simulink model "SF045A_HwAgSysArbn"  (R2013b)
settings: Solver=FixedStepDiscrete  SolverMode=SingleTasking  StartTime=0.0  StopTime=1  FixedStep=.002  RelTol=1e-3
values from neighbouring files (symbols this model uses):
  ARCHGLBPRM_2MILLISEC_SEC_F32 = DataDict.Constant    [SF045A_HwAgSysArbn_DataDict.m]
  ARCHGLBPRM_FLOATZEROTHD_ULS_F32 = DataDict.Constant    [SF045A_HwAgSysArbn_DataDict.m]
  ARCHGLBPRM_PIOVER180_ULS_F32 = DataDict.Constant    [SF045A_HwAgSysArbn_DataDict.m]
  CNVSECTOCNT_ULS_U32 = DataDict.Constant    [SF045A_HwAgSysArbn_DataDict.m]
  CNVTOMILLISEC_MILLISECPERCNT_F32 = DataDict.Constant    [SF045A_HwAgSysArbn_DataDict.m]
  FltInj_f32 = DataDict.Client    [SF045A_HwAgSysArbn_DataDict.m]
  FLTINJ_HWAGSYSARBN_HWAG = DataDict.Constant    [SF045A_HwAgSysArbn_DataDict.m]
  FLTINJ_HWAGSYSARBN_SERLCOMHWAG = DataDict.Constant    [SF045A_HwAgSysArbn_DataDict.m]
  HwAgCorrlnFlt = DataDict.NTC    [SF045A_HwAgSysArbn_DataDict.m]
  HwAgSnsrlsThdExcdd = DataDict.NTC    [SF045A_HwAgSysArbn_DataDict.m]
  HwAgSysArbnHwAgConf1Snsr = DataDict.Calibration    [SF045A_HwAgSysArbn_DataDict.m]
  HwAgSysArbnHwAgConf2Snsr = DataDict.Calibration    [SF045A_HwAgSysArbn_DataDict.m]
  HwAgSysArbnHwAgConfNoSnsr = DataDict.Calibration    [SF045A_HwAgSysArbn_DataDict.m]
  HwAgSysArbnHwAgCorrdCorrlnThd = DataDict.Calibration    [SF045A_HwAgSysArbn_DataDict.m]
  HwAgSysArbnHwAgCorrlnFailDebStep = DataDict.Calibration    [SF045A_HwAgSysArbn_DataDict.m]
  HwAgSysArbnHwAgCorrlnPassDebStep = DataDict.Calibration    [SF045A_HwAgSysArbn_DataDict.m]
  HwAgSysArbnHwAgCorrlnRng = DataDict.Calibration    [SF045A_HwAgSysArbn_DataDict.m]
  HwAgSysArbnHwAgSlewRate = DataDict.Calibration    [SF045A_HwAgSysArbn_DataDict.m]
  HwAgSysArbnHwAgSnsrlsCorrlnThd = DataDict.Calibration    [SF045A_HwAgSysArbn_DataDict.m]
  HwAgSysArbnHwAgSnsrlsKineThd = DataDict.Calibration    [SF045A_HwAgSysArbn_DataDict.m]
  HwAgSysArbnHwAgToMotAgCorrlnElpdTiLim = DataDict.Calibration    [SF045A_HwAgSysArbn_DataDict.m]
  HwAgSysArbnSerlComHwAgCorrdConf = DataDict.Calibration    [SF045A_HwAgSysArbn_DataDict.m]
  HwAgSysArbnSerlComHwAgSnsrlsConf = DataDict.Calibration    [SF045A_HwAgSysArbn_DataDict.m]
  HwAgSysArbnSlewRateTmr = DataDict.Calibration    [SF045A_HwAgSysArbn_DataDict.m]
  HWAGTHD_ULS_FLOAT32 = DataDict.Constant    [SF045A_HwAgSysArbn_DataDict.m]
  INVLDSRC_CNT_S08 = DataDict.Constant    [SF045A_HwAgSysArbn_DataDict.m]
  LRGSLEW_HWDEGPERSEC_F32 = DataDict.Constant    [SF045A_HwAgSysArbn_DataDict.m]
  NODEBSTEP_CNT_U16 = DataDict.Constant    [SF045A_HwAgSysArbn_DataDict.m]
  SLEWINPROGS_CNT_LGC = DataDict.Constant    [SF045A_HwAgSysArbn_DataDict.m]
  SLEWNOTINPROGS_CNT_LGC = DataDict.Constant    [SF045A_HwAgSysArbn_DataDict.m]
  SNSRDATASRCSELD_CNT_S08 = DataDict.Constant    [SF045A_HwAgSysArbn_DataDict.m]
  SNSRLSDATASRCSELD_CNT_S08 = DataDict.Constant    [SF045A_HwAgSysArbn_DataDict.m]
  SysGlbPrmSysKineRat = DataDict.ImprtdCal    [SF045A_HwAgSysArbn_DataDict.m]
  SysGlbPrmTorsBarStfn = DataDict.ImprtdCal    [SF045A_HwAgSysArbn_DataDict.m]
  ZEROTMR_MILLISEC_F32 = DataDict.Constant    [SF045A_HwAgSysArbn_DataDict.m]
undefined symbols (not defined in the file or in its folder): NtcSts1
libraries: NxtrLim x11, simulink x6, NxtrAbslt x6, Fil x3, autosarlib x2
(part 6 of 6)

== system SF045A_HwAgSysArbn/HwAgSysArbn/HwAgSysArbnPer1/HwAgArbn/VldtSnsrlsData/ThdExcdd/Kinematic Integrity/SetNtcSts ==
  note: Note:
      |
      | - "ISO Fault Debounce Design" Simulink block intent to use here for Simulation purpose only. Do not Code this block
  NtcNr : Inport
  NtcStInfo : Inport  Port=2
  NtcSts : Inport  Port=3
  DebStep : Inport  Port=4
  CopyRight2 : Subsystem  Description=|  mask(Copyright Information){none=on}
      | Copyright info block.                                               
      |                                                                     
      | Place copyright information at the top of every subsystem in design.
      mask prompts: none "No parameters"
      mask help: Place copyright information at the top of every subsystem in design.
      mask Display:
      | NxtrConf = 'Nexteer Confidential';
      | 
      | sys = bdroot; %handle for the current model ("system")
      | first = get_param(sys,'Created');
      | if(isempty(first))
      |     first = datestr(now,'yyyy');
      | else
      |     first = first(end-3:end);  %year is last four digits
      | end
      | 
      | last = get_param(sys,'LastModifiedDate');
      | if isempty(last)
      |     last = datestr(now,'yyyy');
      | else
      |     last = last(end-3:end);
      | end
      | 
      | if strcmp(first,last)
      |     fprintf('%s -- Copyright %s Nexteer',NxtrConf,first)
      | else
      |     fprintf('%s -- %s%s- %s Nexteer',NxtrConf,char(169),first,last)
      | end
  Data Store Write : DataStoreWrite  DataStoreName=NtcQlfr
  Data Store Write1 : DataStoreWrite  DataStoreName=NtcQlfrHwAgSnsrlsThdExcd
  Data Store Write2 : DataStoreWrite  DataStoreName=NtcStInfoHwAgSnsrlsThdExcd
  Data Store Write3 : DataStoreWrite  DataStoreName=NtcStsHwAgSnsrlsThdExcd
  Data Type Conversion : DataTypeConversion  OutDataTypeStr=Enum: SigQlfr1
  Data Type Conversion1 : DataTypeConversion  OutDataTypeStr=uint8
  Ground : Ground
  ISO Fault Debounce Design : Stateflow chart  TreatAsAtomicUnit=on
      settings: AttributesFormatString=|
      | Simulation Purpose Only.
      | Do Not Code this block
      | Diagnostic Manager Owns this requirement
  Terminator : Terminator
  Terminator1 : Terminator
  wires:
  Data Type Conversion1/1 -> Data Store Write2/1
  NtcStInfo/1 -> Terminator1/1, Data Type Conversion1/1
  NtcSts/1 -> ISO Fault Debounce Design/1(NtcSts), Data Store Write3/1
  Data Type Conversion/1 -> Data Store Write/1, Data Store Write1/1
  Ground/1 -> ISO Fault Debounce Design/3(SvcClr)
  ISO Fault Debounce Design/1(Qualifier) -> Data Type Conversion/1
  DebStep/1 -> ISO Fault Debounce Design/2(DebStep)
  NtcNr/1 -> Terminator/1

== system SF045A_HwAgSysArbn/HwAgSysArbn/HwAgSysArbnPer1/HwAgArbn/HwAgVelSeriCom/ChkCorrln/SetCorrlFltNtc/SetCorrlFltNtc/SetNtcSts ==
  note: Note:
      |
      | - "ISO Fault Debounce Design" Simulink block intent to use here for Simulation purpose only. Do not Code this block
  NtcNr : Inport
  NtcStInfo : Inport  Port=2
  NtcSts : Inport  Port=3
  DebStep : Inport  Port=4
  CopyRight2 : Subsystem  Description=|  mask(Copyright Information){none=on}
      | Copyright info block.                                               
      |                                                                     
      | Place copyright information at the top of every subsystem in design.
      mask prompts: none "No parameters"
      mask help: Place copyright information at the top of every subsystem in design.
      mask Display:
      | NxtrConf = 'Nexteer Confidential';
      | 
      | sys = bdroot; %handle for the current model ("system")
      | first = get_param(sys,'Created');
      | if(isempty(first))
      |     first = datestr(now,'yyyy');
      | else
      |     first = first(end-3:end);  %year is last four digits
      | end
      | 
      | last = get_param(sys,'LastModifiedDate');
      | if isempty(last)
      |     last = datestr(now,'yyyy');
      | else
      |     last = last(end-3:end);
      | end
      | 
      | if strcmp(first,last)
      |     fprintf('%s -- Copyright %s Nexteer',NxtrConf,first)
      | else
      |     fprintf('%s -- %s%s- %s Nexteer',NxtrConf,char(169),first,last)
      | end
  Data Store Write : DataStoreWrite  DataStoreName=NtcQlfr
  Data Store Write1 : DataStoreWrite  DataStoreName=NtcQlfrHwAgToMotAgCorrln
  Data Store Write2 : DataStoreWrite  DataStoreName=NtcStInfoHwAgToMotAgCorrln
  Data Store Write3 : DataStoreWrite  DataStoreName=NtcStsHwAgToMotAgCorrln
  Data Type Conversion : DataTypeConversion  OutDataTypeStr=Enum: SigQlfr1
  Data Type Conversion1 : DataTypeConversion  OutDataTypeStr=uint8
  Ground : Ground
  ISO Fault Debounce Design : Stateflow chart  TreatAsAtomicUnit=on
      settings: AttributesFormatString=|
      | Simulation Purpose Only.
      | Do Not Code this block
      | Diagnostic Manager Owns this requirement
  Terminator : Terminator
  Terminator1 : Terminator
  wires:
  Data Type Conversion1/1 -> Data Store Write2/1
  NtcStInfo/1 -> Terminator1/1, Data Type Conversion1/1
  NtcSts/1 -> ISO Fault Debounce Design/1(NtcSts), Data Store Write3/1
  Data Type Conversion/1 -> Data Store Write/1, Data Store Write1/1
  Ground/1 -> ISO Fault Debounce Design/3(SvcClr)
  ISO Fault Debounce Design/1(Qualifier) -> Data Type Conversion/1
  DebStep/1 -> ISO Fault Debounce Design/2(DebStep)
  NtcNr/1 -> Terminator/1

== system SF045A_HwAgSysArbn/HwAgSysArbn/HwAgSysArbnPer1/HwAgArbn/HwAgVelSeriCom/ChkCorrln/SetNtcPass/GetRefTmr100MicroSec32bit/CopyRight2 ==

== system SF045A_HwAgSysArbn/HwAgSysArbn/HwAgSysArbnPer1/HwAgArbn/HwAgVelSeriCom/ChkCorrln/SetNtcPass/SetNtcPass/SetNtcSts ==
  note: Note:
      |
      | - "ISO Fault Debounce Design" Simulink block intent to use here for Simulation purpose only. Do not Code this block
  NtcNr : Inport
  NtcStInfo : Inport  Port=2
  NtcSts : Inport  Port=3
  DebStep : Inport  Port=4
  CopyRight2 : Subsystem  Description=|  mask(Copyright Information){none=on}
      | Copyright info block.                                               
      |                                                                     
      | Place copyright information at the top of every subsystem in design.
      mask prompts: none "No parameters"
      mask help: Place copyright information at the top of every subsystem in design.
      mask Display:
      | NxtrConf = 'Nexteer Confidential';
      | 
      | sys = bdroot; %handle for the current model ("system")
      | first = get_param(sys,'Created');
      | if(isempty(first))
      |     first = datestr(now,'yyyy');
      | else
      |     first = first(end-3:end);  %year is last four digits
      | end
      | 
      | last = get_param(sys,'LastModifiedDate');
      | if isempty(last)
      |     last = datestr(now,'yyyy');
      | else
      |     last = last(end-3:end);
      | end
      | 
      | if strcmp(first,last)
      |     fprintf('%s -- Copyright %s Nexteer',NxtrConf,first)
      | else
      |     fprintf('%s -- %s%s- %s Nexteer',NxtrConf,char(169),first,last)
      | end
  Data Store Write : DataStoreWrite  DataStoreName=NtcQlfr
  Data Store Write1 : DataStoreWrite  DataStoreName=NtcQlfrHwAgToMotAgCorrln
  Data Store Write2 : DataStoreWrite  DataStoreName=NtcStInfoHwAgToMotAgCorrln
  Data Store Write3 : DataStoreWrite  DataStoreName=NtcStsHwAgToMotAgCorrln
  Data Type Conversion : DataTypeConversion  OutDataTypeStr=Enum: SigQlfr1
  Data Type Conversion1 : DataTypeConversion  OutDataTypeStr=uint8
  Ground : Ground
  ISO Fault Debounce Design : Stateflow chart  TreatAsAtomicUnit=on
      settings: AttributesFormatString=|
      | Simulation Purpose Only.
      | Do Not Code this block
      | Diagnostic Manager Owns this requirement
  Terminator : Terminator
  Terminator1 : Terminator
  wires:
  NtcNr/1 -> Terminator/1
  DebStep/1 -> ISO Fault Debounce Design/2(DebStep)
  ISO Fault Debounce Design/1(Qualifier) -> Data Type Conversion/1
  Ground/1 -> ISO Fault Debounce Design/3(SvcClr)
  Data Type Conversion/1 -> Data Store Write1/1, Data Store Write/1
  NtcSts/1 -> Data Store Write3/1, ISO Fault Debounce Design/1(NtcSts)
  NtcStInfo/1 -> Data Type Conversion1/1, Terminator1/1
  Data Type Conversion1/1 -> Data Store Write2/1

== system SF045A_HwAgSysArbn/HwAgSysArbn/HwAgSysArbnPer1/HwAgArbn/HwAgVelSeriCom/SnsrlsDataToSerlCom/GetTiSpan100MicroSec32bit/No wrapping/CopyRight2 ==

== system SF045A_HwAgSysArbn/HwAgSysArbn/HwAgSysArbnPer1/HwAgArbn/HwAgVelSeriCom/SnsrlsDataToSerlCom/GetTiSpan100MicroSec32bit/Wrapping/CopyRight2 ==

== system SF045A_HwAgSysArbn/HwAgSysArbn/HwAgSysArbnPer1/HwAgArbn/TestHwAgSrcChg/ApplyRateLim/GetTiSpan100MicroSec32bit/No wrapping/CopyRight2 ==

== system SF045A_HwAgSysArbn/HwAgSysArbn/HwAgSysArbnPer1/HwAgArbn/TestHwAgSrcChg/ApplyRateLim/GetTiSpan100MicroSec32bit/Wrapping/CopyRight2 ==

== system SF045A_HwAgSysArbn/HwAgSysArbn/HwAgSysArbnPer1/HwAgArbn/VldtSnsrlsData/ThdExcdd/Kinematic Integrity/SetNtcSts/CopyRight2 ==

== system SF045A_HwAgSysArbn/HwAgSysArbn/HwAgSysArbnPer1/HwAgArbn/HwAgVelSeriCom/ChkCorrln/SetCorrlFltNtc/SetCorrlFltNtc/SetNtcSts/CopyRight2 ==

== system SF045A_HwAgSysArbn/HwAgSysArbn/HwAgSysArbnPer1/HwAgArbn/HwAgVelSeriCom/ChkCorrln/SetNtcPass/SetNtcPass/SetNtcSts/CopyRight2 ==

== stateflow chart SF045A_HwAgSysArbn/HwAgSysArbn/HwAgSysArbnPer1/HwAgArbn/HwAgVelSeriCom/ChkCorrln/SetNtcPass/SetNtcPass/SetNtcSts/ISO Fault Debounce Design ==
  note: NTCSTS_PASSD           (0)
      | NTCSTS_FAILD             (1)
      | NTCSTS_PREPASSD   (2)
      | NTCSTS_PREFAILD     (3)
      |
      | SIGQLFR_NORES        (0)
      | SIGQLFR_PASSD         (1)
      | SIGQLFR_FAILD           (2)
  note: Pass Loop
  note: Fail Loop
  note: 
  (default) -> (junction 89)
  (junction 89) -> (junction 95) [order 1] : [NtcSts ==3]
  (junction 89) -> (junction 93) [order 2] : [NtcSts ==2]
  (junction 89) -> (junction 141) [order 3] : [NtcSts ==1]
      | { ErrAcc = 32767;
      | Qualifier =2;
      |  }
  (junction 89) -> (junction 141) [order 4] : [NtcSts ==0]
      | { ErrAcc = -32768;
      | Qualifier=1;
      | }
  (junction 95) -> (junction 103) [order 2]
  (junction 95) -> (junction 111) [order 1] : [ErrAcc <=0]
      | {ErrAcc = DebStep;}
  (junction 93) -> (junction 123) [order 2] : {
      | ErrAcc = ErrAcc - DebStep;
      | }
  (junction 93) -> (junction 123) [order 1] : [(ErrAcc - DebStep) <= -32768]
      | { ErrAcc = -32768;
      | Qualifier=1;
      | }
  (junction 103) -> (junction 111) [order 1] : [(ErrAcc + DebStep) <32767]
      | {ErrAcc = ErrAcc + DebStep;}
  (junction 103) -> (junction 111) [order 2] : {ErrAcc = 32767;
      | Qualifier =2;}
  (junction 123) -> (junction 141)
  (junction 111) -> (junction 141)
  (junction 141) -> (junction 159) [order 2] : {ErrAcc = 0;
      | Qualifier =0;
      | }
  (junction 141) -> (junction 159) [order 1] : [SvcClr ==0]
  data: NtcSts input Enum: NtcSts1; Qualifier output uint8; DebStep input uint16; ErrAcc local single; SvcClr input

== stateflow chart SF045A_HwAgSysArbn/HwAgSysArbn/HwAgSysArbnPer1/HwAgArbn/HwAgVelSeriCom/ChkCorrln/SetCorrlFltNtc/SetCorrlFltNtc/SetNtcSts/ISO Fault Debounce Design ==
  note: NTCSTS_PASSD           (0)
      | NTCSTS_FAILD             (1)
      | NTCSTS_PREPASSD   (2)
      | NTCSTS_PREFAILD     (3)
      |
      | SIGQLFR_NORES        (0)
      | SIGQLFR_PASSD         (1)
      | SIGQLFR_FAILD           (2)
  note: Pass Loop
  note: Fail Loop
  note: 
  (default) -> (junction 89)
  (junction 89) -> (junction 95) [order 1] : [NtcSts ==3]
  (junction 89) -> (junction 93) [order 2] : [NtcSts ==2]
  (junction 89) -> (junction 141) [order 3] : [NtcSts ==1]
      | { ErrAcc = 32767;
      | Qualifier =2;
      |  }
  (junction 89) -> (junction 141) [order 4] : [NtcSts ==0]
      | { ErrAcc = -32768;
      | Qualifier=1;
      | }
  (junction 95) -> (junction 103) [order 2]
  (junction 95) -> (junction 111) [order 1] : [ErrAcc <=0]
      | {ErrAcc = DebStep;}
  (junction 93) -> (junction 123) [order 2] : {
      | ErrAcc = ErrAcc - DebStep;
      | }
  (junction 93) -> (junction 123) [order 1] : [(ErrAcc - DebStep) <= -32768]
      | { ErrAcc = -32768;
      | Qualifier=1;
      | }
  (junction 103) -> (junction 111) [order 1] : [(ErrAcc + DebStep) <32767]
      | {ErrAcc = ErrAcc + DebStep;}
  (junction 103) -> (junction 111) [order 2] : {ErrAcc = 32767;
      | Qualifier =2;}
  (junction 123) -> (junction 141)
  (junction 111) -> (junction 141)
  (junction 141) -> (junction 159) [order 2] : {ErrAcc = 0;
      | Qualifier =0;
      | }
  (junction 141) -> (junction 159) [order 1] : [SvcClr ==0]
  data: NtcSts input Enum: NtcSts1; Qualifier output uint8; DebStep input uint16; ErrAcc local single; SvcClr input

== stateflow chart SF045A_HwAgSysArbn/HwAgSysArbn/HwAgSysArbnInit1/Kinematic Integrity/SetNtcSts/ISO Fault Debounce Design ==
  note: NTCSTS_PASSD           (0)
      | NTCSTS_FAILD             (1)
      | NTCSTS_PREPASSD   (2)
      | NTCSTS_PREFAILD     (3)
      |
      | SIGQLFR_NORES        (0)
      | SIGQLFR_PASSD         (1)
      | SIGQLFR_FAILD           (2)
  note: Pass Loop
  note: Fail Loop
  note: 
  (default) -> (junction 89)
  (junction 89) -> (junction 95) [order 1] : [NtcSts ==3]
  (junction 89) -> (junction 93) [order 2] : [NtcSts ==2]
  (junction 89) -> (junction 141) [order 3] : [NtcSts ==1]
      | { ErrAcc = 32767;
      | Qualifier =2;
      |  }
  (junction 89) -> (junction 141) [order 4] : [NtcSts ==0]
      | { ErrAcc = -32768;
      | Qualifier=1;
      | }
  (junction 95) -> (junction 103) [order 2]
  (junction 95) -> (junction 111) [order 1] : [ErrAcc <=0]
      | {ErrAcc = DebStep;}
  (junction 93) -> (junction 123) [order 2] : {
      | ErrAcc = ErrAcc - DebStep;
      | }
  (junction 93) -> (junction 123) [order 1] : [(ErrAcc - DebStep) <= -32768]
      | { ErrAcc = -32768;
      | Qualifier=1;
      | }
  (junction 103) -> (junction 111) [order 1] : [(ErrAcc + DebStep) <32767]
      | {ErrAcc = ErrAcc + DebStep;}
  (junction 103) -> (junction 111) [order 2] : {ErrAcc = 32767;
      | Qualifier =2;}
  (junction 123) -> (junction 141)
  (junction 111) -> (junction 141)
  (junction 141) -> (junction 159) [order 2] : {ErrAcc = 0;
      | Qualifier =0;
      | }
  (junction 141) -> (junction 159) [order 1] : [SvcClr ==0]
  data: NtcSts input Enum: NtcSts1; Qualifier output uint8; DebStep input uint16; ErrAcc local single; SvcClr input

== stateflow chart SF045A_HwAgSysArbn/HwAgSysArbn/HwAgSysArbnPer1/HwAgArbn/VldtSnsrlsData/ThdExcdd/Kinematic Integrity/SetNtcSts/ISO Fault Debounce Design ==
  note: NTCSTS_PASSD           (0)
      | NTCSTS_FAILD             (1)
      | NTCSTS_PREPASSD   (2)
      | NTCSTS_PREFAILD     (3)
      |
      | SIGQLFR_NORES        (0)
      | SIGQLFR_PASSD         (1)
      | SIGQLFR_FAILD           (2)
  note: Pass Loop
  note: Fail Loop
  note: 
  (default) -> (junction 89)
  (junction 89) -> (junction 95) [order 1] : [NtcSts ==3]
  (junction 89) -> (junction 93) [order 2] : [NtcSts ==2]
  (junction 89) -> (junction 141) [order 3] : [NtcSts ==1]
      | { ErrAcc = 32767;
      | Qualifier =2;
      |  }
  (junction 89) -> (junction 141) [order 4] : [NtcSts ==0]
      | { ErrAcc = -32768;
      | Qualifier=1;
      | }
  (junction 95) -> (junction 103) [order 2]
  (junction 95) -> (junction 111) [order 1] : [ErrAcc <=0]
      | {ErrAcc = DebStep;}
  (junction 93) -> (junction 123) [order 2] : {
      | ErrAcc = ErrAcc - DebStep;
      | }
  (junction 93) -> (junction 123) [order 1] : [(ErrAcc - DebStep) <= -32768]
      | { ErrAcc = -32768;
      | Qualifier=1;
      | }
  (junction 103) -> (junction 111) [order 1] : [(ErrAcc + DebStep) <32767]
      | {ErrAcc = ErrAcc + DebStep;}
  (junction 103) -> (junction 111) [order 2] : {ErrAcc = 32767;
      | Qualifier =2;}
  (junction 123) -> (junction 141)
  (junction 111) -> (junction 141)
  (junction 141) -> (junction 159) [order 2] : {ErrAcc = 0;
      | Qualifier =0;
      | }
  (junction 141) -> (junction 159) [order 1] : [SvcClr ==0]
  data: NtcSts input Enum: NtcSts1; Qualifier output uint8; DebStep input uint16; ErrAcc local single; SvcClr input
